simulink model "rocketSim_externalValues"  (R2020b)
settings: Solver=FixedStepAuto  StartTime=0.0  StopTime=time(end)  RelTol=1e-3
libraries: vrlib x3
settings Model: Creator=bean657  LastModifiedBy=Andreas

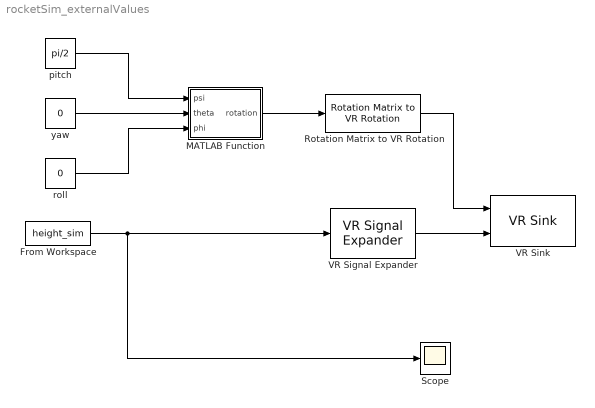
== system rocketSim_externalValues ==
  From Workspace : FromWorkspace  VariableName=height_sim
  MATLAB Function : MATLAB Function  TreatAsAtomicUnit=on
  Rotation Matrix to VR Rotation : vrlib/Utilities/Rotation Matrix to VR Rotation  maxzero=1e-12
      settings: SourceProductBaseCode=SL
  Scope : Scope
  VR Signal Expander : vrlib/VR Signal Expander  outwidth=3  outidx=[2]
  VR Sink : vrlib/VR Sink  InstantiateOnLoad=on  SampleTime=0.1  ViewEnable=on  RemoteChange=off  RemoteView=off  FieldsWritten=Shuttle.rotation.4.1.1.double#Shuttle.translation.3.1.1.double  WorldFileName=rocketWorld.x3d  AutoView=off  VideoDimensions=[]  AllowVariableSize=off
  pitch : Constant  Value=pi/2
  roll : Constant  Value=0
  yaw : Constant  Value=0
  wires:
  VR Signal Expander/1 -> VR Sink/2
  MATLAB Function/1(rotation) -> Rotation Matrix to VR Rotation/1
  pitch/1 -> MATLAB Function/1(psi)
  yaw/1 -> MATLAB Function/2(theta)
  roll/1 -> MATLAB Function/3(phi)
  Rotation Matrix to VR Rotation/1 -> VR Sink/1
  From Workspace/1 -> Scope/1, VR Signal Expander/1

== matlab function rocketSim_externalValues/MATLAB Function ==
  data: psi input; rotation output; theta input; phi input
function rotation = fcn(psi,theta,phi)%yaw pitch roll

%yaw matrix
R3   = [ cos(psi) sin(psi) 0; 
             -sin(psi) cos(psi) 0; 
             0 0 1];
%pitch matrix
R2   = [cos(theta) 0 -sin(theta); 
        0  1           0; 
        sin(theta) 0  cos(theta)];
%roll matrix         
R1    = [1        0          0; 
         0  cos(phi)  sin(phi);
         0 -sin(phi)  cos(phi)];
         
         rotation = R1 * R2 * R3;
end
